simulink model "ModeloBalancin_Discreto"  (R2024a)
settings: Solver=VariableStepAuto  StartTime=0.0  StopTime=10.0  RelTol=1e-3
undefined symbols (not defined in the file): betaF, g, J, Kf, Lb, Lm, m_b, m_m
libraries: simulink_extras x1
settings Model: Creator=Cami  LastModifiedBy=alfar

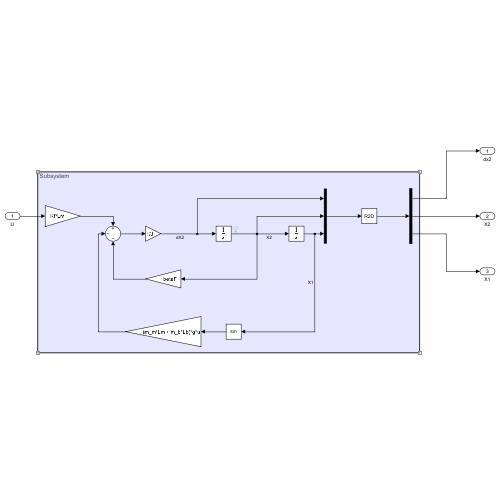
[thumbnail: Simulink's stored preview of the top-level diagram]
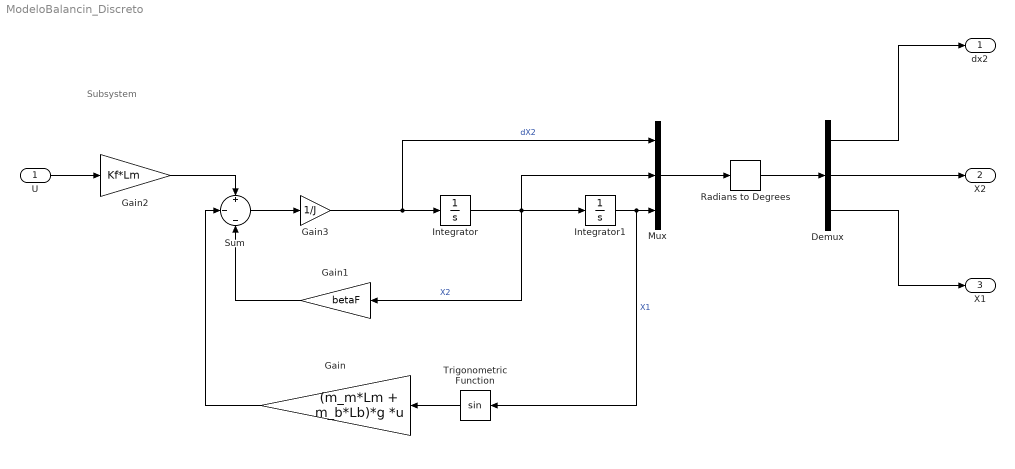
== system ModeloBalancin_Discreto ==
  note: Subsystem
  U : Inport
  Demux : Demux  Outputs=3
  Gain : Gain  Gain=(m_m*Lm + m_b*Lb)*g  Multiplication=Matrix(K*u)
  Gain1 : Gain  Gain=betaF
  Gain2 : Gain  Gain=Kf*Lm
  Gain3 : Gain  Gain=1/J
  Integrator : Integrator
  Integrator1 : Integrator
  Mux : Mux  Inputs=3
  Radians to Degrees : simulink_extras/Transformations/Radians to Degrees
  Sum : Sum  Inputs=+|-|-
  Trigonometric Function : Trigonometry
  dx2 : Outport
  X2 : Outport  Port=2
  X1 : Outport  Port=3
  wires:
  U/1 -> Gain2/1
  Radians to Degrees/1 -> Demux/1
  Gain/1 -> Sum/2
  Demux/1 -> dx2/1
  Gain2/1 -> Sum/1
  Mux/1 -> Radians to Degrees/1
  Gain3/1 -> Mux/1, Integrator/1  "dX2"
  Demux/2 -> X2/1
  Integrator1/1 -> Trigonometric Function/1, Mux/3  "X1"
  Trigonometric Function/1 -> Gain/1
  Demux/3 -> X1/1
  Gain1/1 -> Sum/3
  Sum/1 -> Gain3/1
  Integrator/1 -> Mux/2, Gain1/1, Integrator1/1  "X2"
